simulink model "IEEE30_case"  (R2024b)
settings: Solver=FixedStepAuto  StartTime=0  StopTime=5  FixedStep=1e-7  RelTol=1e-3
values from neighbouring files (symbols this model uses):
  GFL_DFIG_7_C_bus = 0.08    [IEEE30_case_parameters.m]
  GFL_DFIG_7_D_mutual = 2.500000e+3    (= 2500)    [IEEE30_case_parameters.m]
  GFL_DFIG_7_f0 = 60    [IEEE30_case_parameters.m]
  GFL_DFIG_7_gPLLi = 3200    [IEEE30_case_parameters.m]
  GFL_DFIG_7_gPLLp = 650    [IEEE30_case_parameters.m]
  GFL_DFIG_7_H_WT = 0.4    [IEEE30_case_parameters.m]
  GFL_DFIG_7_Hg = 0.8    [IEEE30_case_parameters.m]
  GFL_DFIG_7_Igq_ref = 0    [IEEE30_case_parameters.m]
  GFL_DFIG_7_Ird_ref = 704.45696    [IEEE30_case_parameters.m]
  GFL_DFIG_7_KI_V = -300000    [IEEE30_case_parameters.m]
  GFL_DFIG_7_KP_V = -1000    [IEEE30_case_parameters.m]
  GFL_DFIG_7_Ksh = 1.254300e+4    (= 12543)    [IEEE30_case_parameters.m]
  GFL_DFIG_7_Lg = 0.000483    [IEEE30_case_parameters.m]
  GFL_DFIG_7_Lm_pu = 4    [IEEE30_case_parameters.m]
  GFL_DFIG_7_N = 100    [IEEE30_case_parameters.m]
  GFL_DFIG_7_p = 2    [IEEE30_case_parameters.m]
  GFL_DFIG_7_Pitch = 0    [IEEE30_case_parameters.m]
  GFL_DFIG_7_R = 44    [IEEE30_case_parameters.m]
  GFL_DFIG_7_Rg = 2.000000e-5    (= 2e-05)    [IEEE30_case_parameters.m]
  GFL_DFIG_7_rho = 1.225    [IEEE30_case_parameters.m]
  GFL_DFIG_7_rPLLi = 4500    [IEEE30_case_parameters.m]
  GFL_DFIG_7_rPLLp = 620    [IEEE30_case_parameters.m]
  GFL_DFIG_7_Rs_pu = 0.011    [IEEE30_case_parameters.m]
  GFL_DFIG_7_Sbase = 2.000000e+6    (= 2000000)    [IEEE30_case_parameters.m]
  GFL_DFIG_7_ugq_ref = 0    [IEEE30_case_parameters.m]
  GFL_DFIG_7_usd_ref = 0    [IEEE30_case_parameters.m]
  GFL_DFIG_7_Vbase = 690    [IEEE30_case_parameters.m]
  GFL_DFIG_7_Vdc_ref = 1200    [IEEE30_case_parameters.m]
  GFL_DFIG_7_wind = 12    [IEEE30_case_parameters.m]
  GFL_DFIG_7_wm_ref = 518.184209    [IEEE30_case_parameters.m]
  SG_D_13_D = 0.01056    [IEEE30_case_parameters.m]
  SG_D_13_EnableSaturation = 0    [IEEE30_case_parameters.m]
  SG_D_13_f0 = 60    [IEEE30_case_parameters.m]
  SG_D_13_H = 7.5    [IEEE30_case_parameters.m]
  SG_D_13_K_A = 20    [IEEE30_case_parameters.m]
  SG_D_13_K_E = 1.000000e+1    (= 10)    [IEEE30_case_parameters.m]
  SG_D_13_K_F = 2.363    [IEEE30_case_parameters.m]
  SG_D_13_K_s = 0.5    [IEEE30_case_parameters.m]
  SG_D_13_R_a = 0.001088    [IEEE30_case_parameters.m]
  SG_D_13_S_A = 1    [IEEE30_case_parameters.m]
  SG_D_13_S_B = 0.103    [IEEE30_case_parameters.m]
  SG_D_13_S_N = 10.659857    [IEEE30_case_parameters.m]
  SG_D_13_SpeedPara = 200    [IEEE30_case_parameters.m]
  SG_D_13_T_0 = 0.370163    [IEEE30_case_parameters.m]
  SG_D_13_T_1 = 0.3    [IEEE30_case_parameters.m]
  SG_D_13_T_2 = 0.05    [IEEE30_case_parameters.m]
  SG_D_13_T_3 = 0.02    [IEEE30_case_parameters.m]
  SG_D_13_T_4 = 0.005    [IEEE30_case_parameters.m]
  SG_D_13_T_A = 0.02    [IEEE30_case_parameters.m]
  SG_D_13_T_dd = 8.000000e+0    (= 8)    [IEEE30_case_parameters.m]
  SG_D_13_T_ddd = 0.04    [IEEE30_case_parameters.m]
  SG_D_13_T_E = 0.314    [IEEE30_case_parameters.m]
  SG_D_13_T_F = 0.35    [IEEE30_case_parameters.m]
  SG_D_13_T_qd = 0.8    [IEEE30_case_parameters.m]
  SG_D_13_T_qdd = 0.02    [IEEE30_case_parameters.m]
  SG_D_13_T_speed = 0.1    [IEEE30_case_parameters.m]
  SG_D_13_T_w = 0.5    [IEEE30_case_parameters.m]
  SG_D_13_V_ref = 1.696619    [IEEE30_case_parameters.m]
  SG_D_13_w_ref = 376.991118    [IEEE30_case_parameters.m]
  SG_D_13_x_d = 1.9    [IEEE30_case_parameters.m]
  SG_D_13_x_dd = 0.302    [IEEE30_case_parameters.m]
  SG_D_13_x_ddd = 0.204    [IEEE30_case_parameters.m]
  SG_D_13_x_l = 0.05    [IEEE30_case_parameters.m]
  SG_D_13_x_q = 1.3    [IEEE30_case_parameters.m]
  SG_D_13_x_qd = 0.5    [IEEE30_case_parameters.m]
  SG_D_13_x_qdd = 0.3    [IEEE30_case_parameters.m]
  SG_D_1_D = 0.01056    [IEEE30_case_parameters.m]
  SG_D_1_EnableSaturation = 0    [IEEE30_case_parameters.m]
  SG_D_1_f0 = 60    [IEEE30_case_parameters.m]
  SG_D_1_H = 7.5    [IEEE30_case_parameters.m]
  SG_D_1_K_A = 20    [IEEE30_case_parameters.m]
  SG_D_1_K_E = 1.000000e+1    (= 10)    [IEEE30_case_parameters.m]
  SG_D_1_K_F = 2.363    [IEEE30_case_parameters.m]
  SG_D_1_K_s = 0.5    [IEEE30_case_parameters.m]
  SG_D_1_R_a = 0.001088    [IEEE30_case_parameters.m]
  SG_D_1_S_A = 1    [IEEE30_case_parameters.m]
  SG_D_1_S_B = 0.103    [IEEE30_case_parameters.m]
  SG_D_1_S_N = 10.659857    [IEEE30_case_parameters.m]
  SG_D_1_SpeedPara = 200    [IEEE30_case_parameters.m]
  SG_D_1_T_0 = 0.259812    [IEEE30_case_parameters.m]
  SG_D_1_T_1 = 0.3    [IEEE30_case_parameters.m]
  SG_D_1_T_2 = 0.05    [IEEE30_case_parameters.m]
  SG_D_1_T_3 = 0.02    [IEEE30_case_parameters.m]
  SG_D_1_T_4 = 0.005    [IEEE30_case_parameters.m]
  SG_D_1_T_A = 0.02    [IEEE30_case_parameters.m]
  SG_D_1_T_dd = 8.000000e+0    (= 8)    [IEEE30_case_parameters.m]
  SG_D_1_T_ddd = 0.04    [IEEE30_case_parameters.m]
  SG_D_1_T_E = 0.314    [IEEE30_case_parameters.m]
  SG_D_1_T_F = 0.35    [IEEE30_case_parameters.m]
  SG_D_1_T_qd = 0.8    [IEEE30_case_parameters.m]
  SG_D_1_T_qdd = 0.02    [IEEE30_case_parameters.m]
  SG_D_1_T_speed = 0.1    [IEEE30_case_parameters.m]
  SG_D_1_T_w = 0.5    [IEEE30_case_parameters.m]
  SG_D_1_V_ref = 1.544107    [IEEE30_case_parameters.m]
  SG_D_1_w_ref = 376.991118    [IEEE30_case_parameters.m]
  SG_D_1_x_d = 1.9    [IEEE30_case_parameters.m]
  SG_D_1_x_dd = 0.302    [IEEE30_case_parameters.m]
  SG_D_1_x_ddd = 0.204    [IEEE30_case_parameters.m]
  SG_D_1_x_l = 0.05    [IEEE30_case_parameters.m]
  SG_D_1_x_q = 1.3    [IEEE30_case_parameters.m]
  SG_D_1_x_qd = 0.5    [IEEE30_case_parameters.m]
  SG_D_1_x_qdd = 0.3    [IEEE30_case_parameters.m]
  SG_D_22_D = 0.01056    [IEEE30_case_parameters.m]
  SG_D_22_EnableSaturation = 0    [IEEE30_case_parameters.m]
  SG_D_22_f0 = 60    [IEEE30_case_parameters.m]
  SG_D_22_H = 7.5    [IEEE30_case_parameters.m]
  SG_D_22_K_A = 20    [IEEE30_case_parameters.m]
  SG_D_22_K_E = 1.000000e+1    (= 10)    [IEEE30_case_parameters.m]
  SG_D_22_K_F = 2.363    [IEEE30_case_parameters.m]
  SG_D_22_K_s = 0.5    [IEEE30_case_parameters.m]
  SG_D_22_R_a = 0.001088    [IEEE30_case_parameters.m]
  SG_D_22_S_A = 1    [IEEE30_case_parameters.m]
  SG_D_22_S_B = 0.103    [IEEE30_case_parameters.m]
  SG_D_22_S_N = 10.659857    [IEEE30_case_parameters.m]
  SG_D_22_SpeedPara = 200    [IEEE30_case_parameters.m]
  SG_D_22_T_0 = 0.216121    [IEEE30_case_parameters.m]
  SG_D_22_T_1 = 0.3    [IEEE30_case_parameters.m]
  SG_D_22_T_2 = 0.05    [IEEE30_case_parameters.m]
  SG_D_22_T_3 = 0.02    [IEEE30_case_parameters.m]
  SG_D_22_T_4 = 0.005    [IEEE30_case_parameters.m]
  ... (+126 more)
(part 1 of 27)
settings Model: SimulationMode=accelerator  Creator=Greg  LastModifiedBy=Greg
settings DataIOCC: ReturnWorkspaceOutputs=off

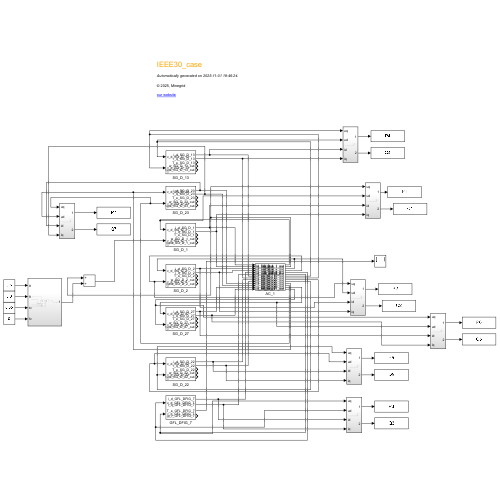
[thumbnail: Simulink's stored preview of the top-level diagram]
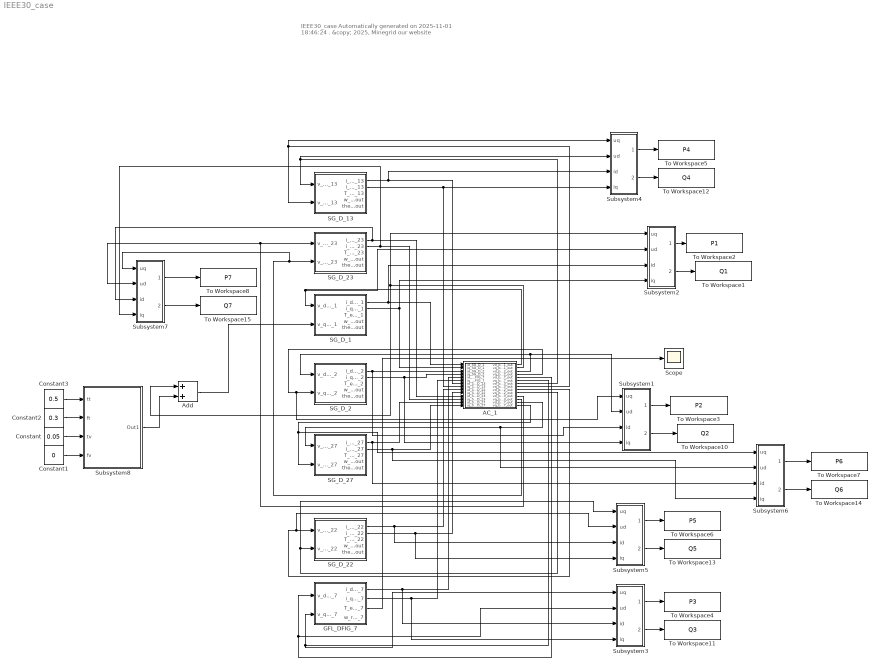
== system IEEE30_case ==
  note: IEEE30_case
      | Automatically generated on 2025-11-01 18:46:24 .
      | &copy; 2025, Minegrid
      | our website
  AC_1 : Subsystem  mask(AC_1){}
      mask help: Parameters Interface of AC_1
  Add : Sum
  Constant : Constant  Value=0.05
  Constant1 : Constant  Value=0
  Constant2 : Constant  Value=0.3
  Constant3 : Constant  Value=0.5
  GFL_DFIG_7 : Subsystem  mask(GFL_DFIG_7){Ird_ref=GFL_DFIG_7_Ird_ref, wm_ref=GFL_DFIG_7_wm_ref, f0=GFL_DFIG_7_f0, Igq_ref=GFL_DFIG_7_Igq_ref, Vdc_ref=GFL_DFIG_7_Vdc_ref, rPLLp=GFL_DFIG_7_rPLLp, rPLLi=GFL_DFIG_7_rPLLi, gPLLp=GFL_DFIG_7_gPLLp, gPLLi=GFL_DFIG_7_gPLLi, Rg=GFL_DFIG_7_Rg, Lg=GFL_DFIG_7_Lg, C_bus=GFL_DFIG_7_C_bus, Hg=GFL_DFIG_7_Hg, D_mutual=GFL_DFIG_7_D_mutual, wind=GFL_DFIG_7_wind, Sbase=GFL_DFIG_7_Sbase, Vbase=GFL_DFIG_7_Vbase, usd_ref=GFL_DFIG_7_usd_ref, ugq_ref=GFL_DFIG_7_ugq_ref, p=GFL_DFIG_7_p, Rs_pu=GFL_DFIG_7_Rs_pu, Lm_pu=GFL_DFIG_7_Lm_pu, rho=GFL_DFIG_7_rho, R=GFL_DFIG_7_R, Pitch=GFL_DFIG_7_Pitch, N=GFL_DFIG_7_N, Ksh=GFL_DFIG_7_Ksh, H_WT=GFL_DFIG_7_H_WT, KP_V=GFL_DFIG_7_KP_V, KI_V=GFL_DFIG_7_KI_V}
      mask help: Parameters Interface of GFL_DFIG_7
  SG_D_1 : Subsystem  mask(SG_D_1){T_0=SG_D_1_T_0, w_ref=SG_D_1_w_ref, V_ref=SG_D_1_V_ref, x_d=SG_D_1_x_d, x_dd=SG_D_1_x_dd, x_ddd=SG_D_1_x_ddd, x_q=SG_D_1_x_q, x_qd=SG_D_1_x_qd, x_qdd=SG_D_1_x_qdd, x_l=SG_D_1_x_l, R_a=SG_D_1_R_a, T_dd=SG_D_1_T_dd, T_ddd=SG_D_1_T_ddd, T_qd=SG_D_1_T_qd, T_qdd=SG_D_1_T_qdd, H=SG_D_1_H, D=SG_D_1_D, SpeedPara=SG_D_1_SpeedPara, K_A=SG_D_1_K_A, EnableSaturation=SG_D_1_EnableSaturation, f0=SG_D_1_f0, T_speed=SG_D_1_T_speed, T_E=SG_D_1_T_E, T_A=SG_D_1_T_A, T_F=SG_D_1_T_F, K_E=SG_D_1_K_E, K_F=SG_D_1_K_F, K_s=SG_D_1_K_s, T_1=SG_D_1_T_1, T_2=SG_D_1_T_2, T_3=SG_D_1_T_3, T_4=SG_D_1_T_4, T_w=SG_D_1_T_w, S_A=SG_D_1_S_A, S_B=SG_D_1_S_B, S_N=SG_D_1_S_N}
      mask help: Parameters Interface of SG_D_1
  SG_D_13 : Subsystem  mask(SG_D_13){T_0=SG_D_13_T_0, w_ref=SG_D_13_w_ref, V_ref=SG_D_13_V_ref, x_d=SG_D_13_x_d, x_dd=SG_D_13_x_dd, x_ddd=SG_D_13_x_ddd, x_q=SG_D_13_x_q, x_qd=SG_D_13_x_qd, x_qdd=SG_D_13_x_qdd, x_l=SG_D_13_x_l, R_a=SG_D_13_R_a, T_dd=SG_D_13_T_dd, T_ddd=SG_D_13_T_ddd, T_qd=SG_D_13_T_qd, T_qdd=SG_D_13_T_qdd, H=SG_D_13_H, D=SG_D_13_D, SpeedPara=SG_D_13_SpeedPara, K_A=SG_D_13_K_A, EnableSaturation=SG_D_13_EnableSaturation, f0=SG_D_13_f0, T_speed=SG_D_13_T_speed, T_E=SG_D_13_T_E, T_A=SG_D_13_T_A, T_F=SG_D_13_T_F, K_E=SG_D_13_K_E, K_F=SG_D_13_K_F, K_s=SG_D_13_K_s, T_1=SG_D_13_T_1, T_2=SG_D_13_T_2, T_3=SG_D_13_T_3, T_4=SG_D_13_T_4, T_w=SG_D_13_T_w, S_A=SG_D_13_S_A, S_B=SG_D_13_S_B, S_N=SG_D_13_S_N}
      mask help: Parameters Interface of SG_D_13
  SG_D_2 : Subsystem  mask(SG_D_2){T_0=SG_D_2_T_0, w_ref=SG_D_2_w_ref, V_ref=SG_D_2_V_ref, x_d=SG_D_2_x_d, x_dd=SG_D_2_x_dd, x_ddd=SG_D_2_x_ddd, x_q=SG_D_2_x_q, x_qd=SG_D_2_x_qd, x_qdd=SG_D_2_x_qdd, x_l=SG_D_2_x_l, R_a=SG_D_2_R_a, T_dd=SG_D_2_T_dd, T_ddd=SG_D_2_T_ddd, T_qd=SG_D_2_T_qd, T_qdd=SG_D_2_T_qdd, H=SG_D_2_H, D=SG_D_2_D, SpeedPara=SG_D_2_SpeedPara, K_A=SG_D_2_K_A, EnableSaturation=SG_D_2_EnableSaturation, f0=SG_D_2_f0, T_speed=SG_D_2_T_speed, T_E=SG_D_2_T_E, T_A=SG_D_2_T_A, T_F=SG_D_2_T_F, K_E=SG_D_2_K_E, K_F=SG_D_2_K_F, K_s=SG_D_2_K_s, T_1=SG_D_2_T_1, T_2=SG_D_2_T_2, T_3=SG_D_2_T_3, T_4=SG_D_2_T_4, T_w=SG_D_2_T_w, S_A=SG_D_2_S_A, S_B=SG_D_2_S_B, S_N=SG_D_2_S_N}
      mask help: Parameters Interface of SG_D_2
  SG_D_22 : Subsystem  mask(SG_D_22){T_0=SG_D_22_T_0, w_ref=SG_D_22_w_ref, V_ref=SG_D_22_V_ref, x_d=SG_D_22_x_d, x_dd=SG_D_22_x_dd, x_ddd=SG_D_22_x_ddd, x_q=SG_D_22_x_q, x_qd=SG_D_22_x_qd, x_qdd=SG_D_22_x_qdd, x_l=SG_D_22_x_l, R_a=SG_D_22_R_a, T_dd=SG_D_22_T_dd, T_ddd=SG_D_22_T_ddd, T_qd=SG_D_22_T_qd, T_qdd=SG_D_22_T_qdd, H=SG_D_22_H, D=SG_D_22_D, SpeedPara=SG_D_22_SpeedPara, K_A=SG_D_22_K_A, EnableSaturation=SG_D_22_EnableSaturation, f0=SG_D_22_f0, T_speed=SG_D_22_T_speed, T_E=SG_D_22_T_E, T_A=SG_D_22_T_A, T_F=SG_D_22_T_F, K_E=SG_D_22_K_E, K_F=SG_D_22_K_F, K_s=SG_D_22_K_s, T_1=SG_D_22_T_1, T_2=SG_D_22_T_2, T_3=SG_D_22_T_3, T_4=SG_D_22_T_4, T_w=SG_D_22_T_w, S_A=SG_D_22_S_A, S_B=SG_D_22_S_B, S_N=SG_D_22_S_N}
      mask help: Parameters Interface of SG_D_22
  SG_D_23 : Subsystem  mask(SG_D_23){T_0=SG_D_23_T_0, w_ref=SG_D_23_w_ref, V_ref=SG_D_23_V_ref, x_d=SG_D_23_x_d, x_dd=SG_D_23_x_dd, x_ddd=SG_D_23_x_ddd, x_q=SG_D_23_x_q, x_qd=SG_D_23_x_qd, x_qdd=SG_D_23_x_qdd, x_l=SG_D_23_x_l, R_a=SG_D_23_R_a, T_dd=SG_D_23_T_dd, T_ddd=SG_D_23_T_ddd, T_qd=SG_D_23_T_qd, T_qdd=SG_D_23_T_qdd, H=SG_D_23_H, D=SG_D_23_D, SpeedPara=SG_D_23_SpeedPara, K_A=SG_D_23_K_A, EnableSaturation=SG_D_23_EnableSaturation, f0=SG_D_23_f0, T_speed=SG_D_23_T_speed, T_E=SG_D_23_T_E, T_A=SG_D_23_T_A, T_F=SG_D_23_T_F, K_E=SG_D_23_K_E, K_F=SG_D_23_K_F, K_s=SG_D_23_K_s, T_1=SG_D_23_T_1, T_2=SG_D_23_T_2, T_3=SG_D_23_T_3, T_4=SG_D_23_T_4, T_w=SG_D_23_T_w, S_A=SG_D_23_S_A, S_B=SG_D_23_S_B, S_N=SG_D_23_S_N}
      mask help: Parameters Interface of SG_D_23
  SG_D_27 : Subsystem  mask(SG_D_27){T_0=SG_D_27_T_0, w_ref=SG_D_27_w_ref, V_ref=SG_D_27_V_ref, x_d=SG_D_27_x_d, x_dd=SG_D_27_x_dd, x_ddd=SG_D_27_x_ddd, x_q=SG_D_27_x_q, x_qd=SG_D_27_x_qd, x_qdd=SG_D_27_x_qdd, x_l=SG_D_27_x_l, R_a=SG_D_27_R_a, T_dd=SG_D_27_T_dd, T_ddd=SG_D_27_T_ddd, T_qd=SG_D_27_T_qd, T_qdd=SG_D_27_T_qdd, H=SG_D_27_H, D=SG_D_27_D, SpeedPara=SG_D_27_SpeedPara, K_A=SG_D_27_K_A, EnableSaturation=SG_D_27_EnableSaturation, f0=SG_D_27_f0, T_speed=SG_D_27_T_speed, T_E=SG_D_27_T_E, T_A=SG_D_27_T_A, T_F=SG_D_27_T_F, K_E=SG_D_27_K_E, K_F=SG_D_27_K_F, K_s=SG_D_27_K_s, T_1=SG_D_27_T_1, T_2=SG_D_27_T_2, T_3=SG_D_27_T_3, T_4=SG_D_27_T_4, T_w=SG_D_27_T_w, S_A=SG_D_27_S_A, S_B=SG_D_27_S_B, S_N=SG_D_27_S_N}
      mask help: Parameters Interface of SG_D_27
  Scope : Scope
  Subsystem1 : Subsystem
  Subsystem2 : Subsystem
  Subsystem3 : Subsystem
  Subsystem4 : Subsystem
  Subsystem5 : Subsystem
  Subsystem6 : Subsystem
  Subsystem7 : Subsystem
  Subsystem8 : Subsystem
  To Workspace1 : ToWorkspace  VariableName=Q1  SampleTime=-1
  To Workspace10 : ToWorkspace  VariableName=Q2  SampleTime=-1
  To Workspace11 : ToWorkspace  VariableName=Q3  SampleTime=-1
  To Workspace12 : ToWorkspace  VariableName=Q4  SampleTime=-1
  To Workspace13 : ToWorkspace  VariableName=Q5  SampleTime=-1
  To Workspace14 : ToWorkspace  VariableName=Q6  SampleTime=-1
  To Workspace15 : ToWorkspace  VariableName=Q7  SampleTime=-1
  To Workspace2 : ToWorkspace  VariableName=P1  SampleTime=-1
  To Workspace3 : ToWorkspace  VariableName=P2  SampleTime=-1
  To Workspace4 : ToWorkspace  VariableName=P3  SampleTime=-1
  To Workspace5 : ToWorkspace  VariableName=P4  SampleTime=-1
  To Workspace6 : ToWorkspace  VariableName=P5  SampleTime=-1
  To Workspace7 : ToWorkspace  VariableName=P6  SampleTime=-1
  To Workspace8 : ToWorkspace  VariableName=P7  SampleTime=-1
  wires:
  SG_D_23/2(i_q_SG_D_23) -> Subsystem7/4(iq), AC_1/12(iq_SG_D_23)
  SG_D_13/1(i_d_SG_D_13) -> Subsystem4/3(id), AC_1/7(id_SG_D_13)
  SG_D_13/2(i_q_SG_D_13) -> Subsystem4/4(iq), AC_1/8(iq_SG_D_13)
  SG_D_23/1(i_d_SG_D_23) -> Subsystem7/3(id), AC_1/11(id_SG_D_23)
  SG_D_2/2(i_q_SG_D_2) -> Subsystem1/4(iq), AC_1/4(iq_SG_D_2)
  SG_D_1/2(i_q_SG_D_1) -> Subsystem2/4(iq), AC_1/2(iq_SG_D_1)
  SG_D_1/1(i_d_SG_D_1) -> Subsystem2/3(id), AC_1/1(id_SG_D_1)
  SG_D_2/1(i_d_SG_D_2) -> Subsystem1/3(id), AC_1/3(id_SG_D_2)
  SG_D_27/1(i_d_SG_D_27) -> Subsystem6/3(id), AC_1/13(id_SG_D_27)
  SG_D_27/2(i_q_SG_D_27) -> Subsystem6/4(iq), AC_1/14(iq_SG_D_27)
  SG_D_22/2(i_q_SG_D_22) -> Subsystem5/4(iq), AC_1/10(iq_SG_D_22)
  SG_D_22/1(i_d_SG_D_22) -> Subsystem5/3(id), AC_1/9(id_SG_D_22)
  AC_1/7(vd_bus_13_out) -> SG_D_13/1(v_d_SG_D_13), Subsystem4/2(ud)
  GFL_DFIG_7/1(i_d_GFL_DFIG_7) -> Subsystem3/3(id), AC_1/5(id_GFL_DFIG_7)
  GFL_DFIG_7/2(i_q_GFL_DFIG_7) -> Subsystem3/4(iq), AC_1/6(iq_GFL_DFIG_7)
  AC_1/3(vd_bus_2_out) -> SG_D_2/1(v_d_SG_D_2), Subsystem1/2(ud)
  AC_1/1(vd_bus_1_out) -> Subsystem2/2(ud), SG_D_1/1(v_d_SG_D_1)
  AC_1/6(vq_bus_7_out) -> GFL_DFIG_7/2(v_q_GFL_DFIG_7), Subsystem3/1(uq)
  AC_1/4(vq_bus_2_out) -> Subsystem1/1(uq), SG_D_2/2(v_q_SG_D_2)
  AC_1/5(vd_bus_7_out) -> GFL_DFIG_7/1(v_d_GFL_DFIG_7), Subsystem3/2(ud)
  AC_1/8(vq_bus_13_out) -> SG_D_13/2(v_q_SG_D_13), Subsystem4/1(uq)
  AC_1/11(vd_bus_23_out) -> SG_D_23/1(v_d_SG_D_23), Subsystem7/2(ud)
  AC_1/9(vd_bus_22_out) -> Subsystem5/2(ud), SG_D_22/1(v_d_SG_D_22)
  AC_1/10(vq_bus_22_out) -> Subsystem5/1(uq), SG_D_22/2(v_q_SG_D_22)
  AC_1/14(vq_bus_27_out) -> SG_D_27/2(v_q_SG_D_27), Subsystem6/1(uq)
  AC_1/12(vq_bus_23_out) -> Subsystem7/1(uq), SG_D_23/2(v_q_SG_D_23)
  AC_1/13(vd_bus_27_out) -> SG_D_27/1(v_d_SG_D_27), Subsystem6/2(ud)
  GFL_DFIG_7/3(T_e_GFL_DFIG_7) -> Scope/1
  Subsystem2/1(Out1) -> To Workspace2/1
  Subsystem2/2(Out2) -> To Workspace1/1
  Subsystem1/1(Out1) -> To Workspace3/1
  Subsystem1/2(Out2) -> To Workspace10/1
  Subsystem3/2(Out2) -> To Workspace11/1
  Subsystem3/1(Out1) -> To Workspace4/1
  Subsystem4/1(Out1) -> To Workspace5/1
  Subsystem4/2(Out2) -> To Workspace12/1
  Subsystem5/1(Out1) -> To Workspace6/1
  Subsystem5/2(Out2) -> To Workspace13/1
  Subsystem6/1(Out1) -> To Workspace7/1
  Subsystem6/2(Out2) -> To Workspace14/1
  Subsystem7/1(Out1) -> To Workspace8/1
  Subsystem7/2(Out2) -> To Workspace15/1
  Constant3/1 -> Subsystem8/1(tt)
  Constant1/1 -> Subsystem8/4(fv)
  Constant/1 -> Subsystem8/3(tv)
  AC_1/2(vq_bus_1_out) -> Add/1, Subsystem2/1(uq)
  Subsystem8/1(Out1) -> Add/2
  Constant2/1 -> Subsystem8/2(ft)
  Add/1 -> SG_D_1/2(v_q_SG_D_1)
